simulink model "Tarea1Ejercicio1SeccionF"  (R2021a)
settings: Solver=VariableStepAuto  StartTime=0.0  StopTime=100  RelTol=1e-3
values from neighbouring files (symbols this model uses):
  A = 3    [Tarea1Parte1SeccionE.m]    (also in Tarea1_Parte1_Todaslassecciones.m; simulink.m)
  g = 9.81    [Tarea1Parte1SeccionE.m]    (also in Tarea1_Parte1_Todaslassecciones.m; Tarea1parte1SeccionD.m; simulink.m)
  K1 = 71.888    [Tarea1Parte1SeccionE.m]    (also in Tarea1_Parte1_Todaslassecciones.m)
  K2 = -10    [Tarea1Parte1SeccionE.m]    (also in Tarea1_Parte1_Todaslassecciones.m)
  Kt = (1/3.3)*100    (= 30.303030303)    [Tarea1Parte1SeccionE.m]    (also in Tarea1_Parte1_Todaslassecciones.m = 0.303; simulink.m)
  Kvc = 0.001    [Tarea1Parte1SeccionE.m]    (also in Tarea1_Parte1_Todaslassecciones.m = 0.1)
  Kvs = 0.001    [Tarea1_Parte1_Todaslassecciones.m]    (also in Tarea1parte1SeccionD.m; simulink.m)
  Qe = 0.6955    [Tarea1_Parte1_Todaslassecciones.m]    (also in simulink.m = (0:0.001:0.1))
  rho = 789    [Tarea1Parte1SeccionE.m]    (also in Tarea1_Parte1_Todaslassecciones.m; Tarea1parte1SeccionD.m; simulink.m)
  T = 215.664    [Tarea1Parte1SeccionE.m]    (also in Tarea1_Parte1_Todaslassecciones.m)
  U = 100    [Tarea1_Parte1_Todaslassecciones.m]
  Uf = U*0.98    (= 98)    [Tarea1_Parte1_Todaslassecciones.m]
  Xvs0 = 0.5    [Tarea1Parte1SeccionE.m]    (also in Tarea1Parte1SeccionF.m; Tarea1_Parte1_Todaslassecciones.m)
settings Model: Creator=Royer  LastModifiedBy=Royer

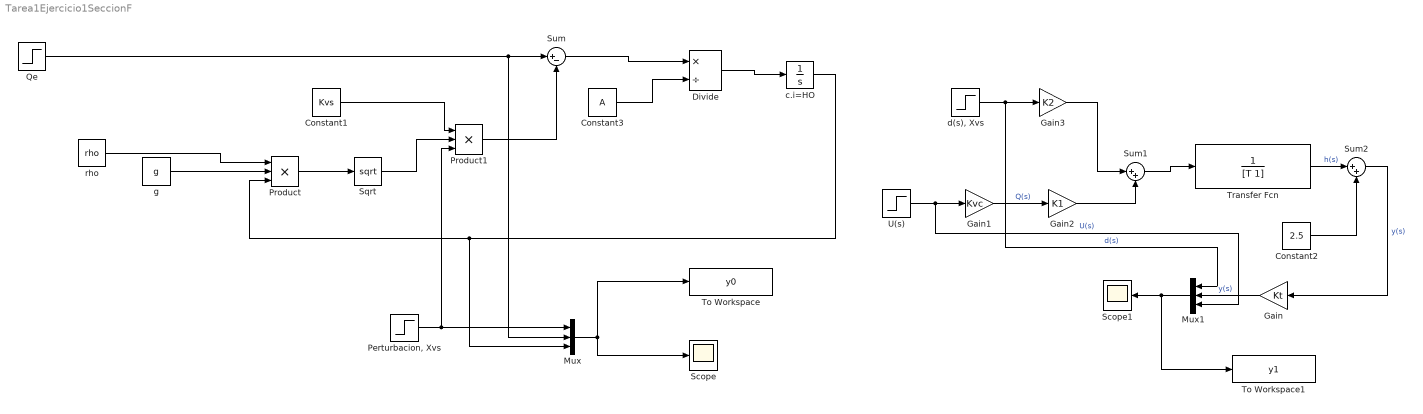
== system Tarea1Ejercicio1SeccionF ==
  Constant1 : Constant  Value=Kvs
  Constant2 : Constant  Value=2.5
  Constant3 : Constant  Value=A
  Divide : Product  Inputs=*/
  Gain : Gain  Gain=Kt
  Gain1 : Gain  Gain=Kvc
  Gain2 : Gain  Gain=K1
  Gain3 : Gain  Gain=K2
  Mux : Mux  Inputs=3
  Mux1 : Mux  Inputs=3
  "Perturbacion, Xvs" : Step  Time=10  Before=Xvs0  After=0.52  SampleTime=0
  Product : Product  Inputs=3
  Product1 : Product  Inputs=3
  Qe : Step  Time=0  Before=Qe  After=Qe-0.02  SampleTime=0
  Scope : Scope
  Scope1 : Scope
  Sqrt : Sqrt  SaturateOnIntegerOverflow=on
  Sum : Sum  Inputs=|+-
  Sum1 : Sum  Inputs=|++
  Sum2 : Sum  Inputs=|++
  To Workspace : ToWorkspace  VariableName=y0  SaveFormat=Timeseries  SampleTime=-1
  To Workspace1 : ToWorkspace  VariableName=y1  SaveFormat=Timeseries  SampleTime=-1
  Transfer Fcn : TransferFcn  Denominator=[T 1]
  U(s) : Step  Before=U  After=Uf  SampleTime=0
  c.i=HO : Integrator  InitialCondition=2.5
  "d(s), Xvs" : Step  Before=Xvs0  SampleTime=0
  g : Constant  Value=g
  rho : Constant  Value=rho
  wires:
  Mux/1 -> Scope/1, To Workspace/1
  Qe/1 -> Sum/1, Mux/2
  Sum/1 -> Divide/1
  c.i=HO/1 -> Product/3, Mux/3
  Divide/1 -> c.i=HO/1
  g/1 -> Product/2
  Product1/1 -> Sum/2
  Sqrt/1 -> Product1/2
  Product/1 -> Sqrt/1
  rho/1 -> Product/1
  Constant1/1 -> Product1/1
  U(s)/1 -> Mux1/3, Gain1/1  "U(s)"
  Gain3/1 -> Sum1/1
  Gain1/1 -> Gain2/1  "Q(s)"
  "d(s), Xvs"/1 -> Mux1/1, Gain3/1  "d(s)"
  Sum1/1 -> Transfer Fcn/1
  Gain2/1 -> Sum1/2
  Transfer Fcn/1 -> Sum2/1  "h(s)"
  Constant2/1 -> Sum2/2
  Sum2/1 -> Gain/1  "y(s)"
  Mux1/1 -> To Workspace1/1, Scope1/1
  Gain/1 -> Mux1/2  "y(s)"
  Constant3/1 -> Divide/2
  "Perturbacion, Xvs"/1 -> Mux/1, Product1/3
